simulink model "sgMdl_BatteryEmulation"  (R2024b)
settings: Solver=FixedStepAuto  StartTime=0.0  StopTime=inf  RelTol=1e-3  EnableMultiTasking=on
libraries: simulink x2, speedgoatlib_PIL x1
Description:
  | Battery Emulation
settings Model: ModifiedByFormat=Speedgoat  SimulationMode=external  ExtModeTrigDuration=100000  Creator=Speedgoat  LastModifiedBy=Speedgoat
settings SolverCC: ConcurrentTasks=on  AlgebraicLoopSolver=TrustRegion  PositivePriorityOrder=on  InsertRTBMode=Never (minimum delay)
settings DataIOCC: SaveFormat=Array  SaveState=on  SignalLoggingName=logsOut
settings OptimizationCC: BlockReduction=off  BooleanDataType=off  OptimizeBlockIOStorage=off  BufferReuse=off  ReuseModelBlockBuffer=off  GlobalBufferReuse=off  ExpressionFolding=off  LocalBlockOutputs=off  InitFltsAndDblsToZero=on  OptimizeDataStoreBuffers=off  BusAssignmentInplaceUpdate=off
settings DebuggingCC: SaveWithParameterizedLinksMsg=none  UnderspecifiedInitializationDetection=Classic  MergeDetectMultiDrivingBlocksExec=none  CheckExecutionContextPreStartOutputMsg=on  SignalResolutionControl=TryResolveAllWithWarning  TasksWithSamePriorityMsg=none  UnconnectedInputMsg=warning  UnconnectedOutputMsg=warning  UnconnectedLineMsg=warning  SFUnexpectedBacktrackingDiag=warning  SFNoUnconditionalDefaultTransitionDiag=warning  SFExecutionAtInitializationDiag=none  ArithmeticOperatorsInVariantConditions=warning
settings HardwareCC: ProdBitPerLong=64  ProdLongLongMode=on  ProdHWDeviceType=Intel->x86-64 (Linux 64)
settings ModelReferenceCC: EnableRefExpFcnMdlSchedulingChecks=on  PropagateSignalLabelsOutOfModel=off
settings SFSimCC: SimUseLocalCustomCode=off  SimTargetLang=C++
settings RTWCC: Description=Speedgoat Real-Time Target Machine  SystemTargetFile=speedgoat.tlc  TemplateMakefile=slrealtime_default_tmf  PostCodeGenCommand=sg.model.build.makeCfg(bdroot, buildInfo);  RTWUseLocalCustomCode=off  Toolchain=Simulink Real-Time Toolchain  BuildConfiguration=Faster Runs  TargetLang=C++  GPUComputeCapability=3.5  DLArmComputeVersion=19.05
settings CodeAppCC: StateflowObjectComments=on
settings SimulinkRealTimeTargetCC: SubcomponentCodeInterfacePackaging=Reusable function  MATLABClassNameForMDSCustomization=Simulink.SoftwareTarget.GRTCustomization  InstructionSetFMA=off  LogToMDFFile=off  SLRTFileLogMaxRuns=10  UseGCCFastMath=on
settings ConfigComp: CovMetricSettings=dw  CovSaveCumulativeToWorkspaceVar=on  CovSaveSingleToWorkspaceVar=on  CovExternalEMLEnable=off  CovSFcnEnable=off  CovBoundaryAbsTol=1.0e-5

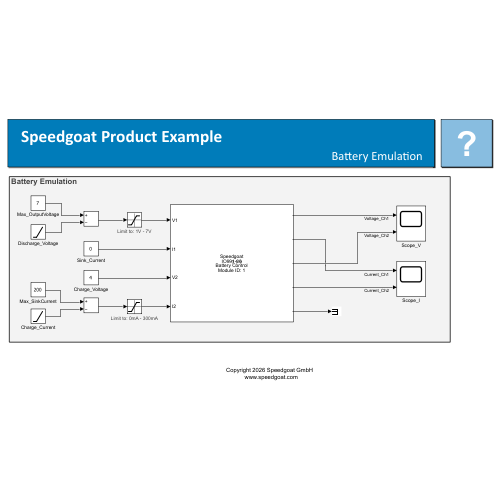
[thumbnail: Simulink's stored preview of the top-level diagram]
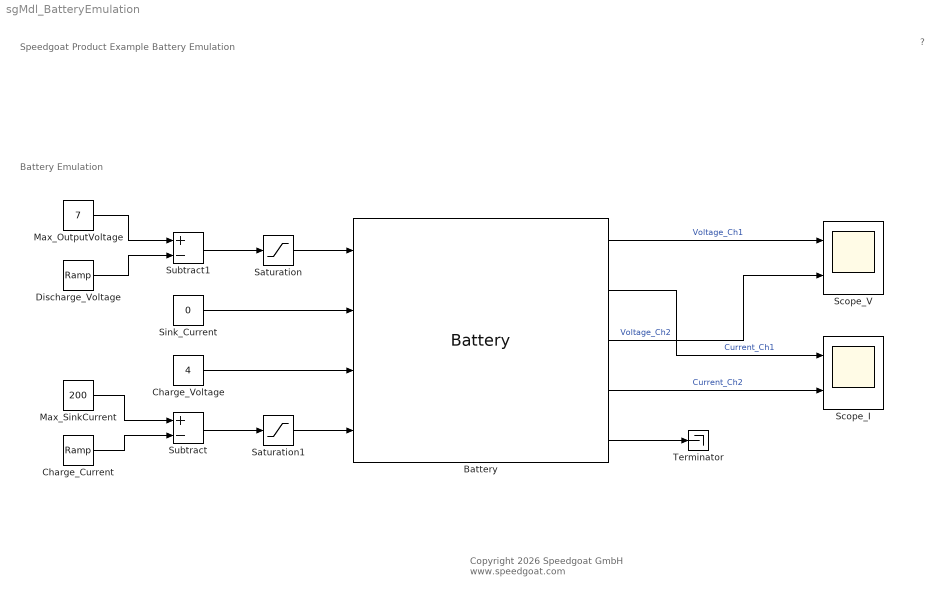
== system sgMdl_BatteryEmulation ==
  note: Battery Emulation
  note: Speedgoat Product Example
      | Battery Emulation
  note: ?
  note: Copyright 2026 Speedgoat GmbH
      |  www.speedgoat.com
  Battery : speedgoatlib_PIL/Battery  id=1  card_type=IO992-06 (6 channels, 0-7V output, 300mA source, 300mA sink)  channel_vector=[1,2]  init_enable_vector=[1]  reset_enable_vector=[0]  init_voltage_vector=[0]  reset_voltage_vector=[1]  init_current_vector=[0]  reset_current_vector=[1]  no_samples=16  conv_time_voltage=540  conv_time_current=540  show_input_enable=off  show_output=on  ts=-1  slot=-1  VendorID=0  SubVendorID=0  DeviceID=0  SubDeviceID=0  category=1  NumCh=0  MinVout=0  MaxVout=0  MinIsink=0  MaxIsink=0
      settings: SourceProductName=Simulink Real-Time: Speedgoat I/O Blockset
  Charge_Current : simulink/Sources/Ramp  slope=30  start=3  InitialOutput=0
  Charge_Voltage : Constant  Value=4  SampleTime=0.1
  Discharge_Voltage : simulink/Sources/Ramp  slope=1  start=3  InitialOutput=1
  Max_OutputVoltage : Constant  Value=7  SampleTime=0.1
  Max_SinkCurrent : Constant  Value=200  SampleTime=0.1
  Saturation : Saturate  UpperLimit=7  LowerLimit=1
      settings: AttributesFormatString=Limit to: %<LowerLimit>V - %<UpperLimit>V
  Saturation1 : Saturate  UpperLimit=300  LowerLimit=0
      settings: AttributesFormatString=Limit to: %<LowerLimit>mA - %<UpperLimit>mA
  Scope_I : Scope  NumInputPorts=2
  Scope_V : Scope  NumInputPorts=2
  Sink_Current : Constant  Value=0  SampleTime=0.1
  Subtract : Sum  Inputs=+-
  Subtract1 : Sum  Inputs=+-
  Terminator : Terminator
  wires:
  Sink_Current/1 -> Battery/2
  Charge_Voltage/1 -> Battery/3
  Battery/1 -> Scope_V/1  "Voltage_Ch1"
  Battery/4 -> Scope_I/2  "Current_Ch2"
  Battery/5 -> Terminator/1
  Subtract/1 -> Saturation1/1
  Charge_Current/1 -> Subtract/2
  Max_SinkCurrent/1 -> Subtract/1
  Subtract1/1 -> Saturation/1
  Max_OutputVoltage/1 -> Subtract1/1
  Discharge_Voltage/1 -> Subtract1/2
  Saturation/1 -> Battery/1
  Saturation1/1 -> Battery/4
  Battery/3 -> Scope_V/2  "Voltage_Ch2"
  Battery/2 -> Scope_I/1  "Current_Ch1"
